simulink model "DSB_AMwithAWGN"  (R2018a)
settings: Solver=VariableStepAuto  StartTime=0.0  StopTime=0.005  RelTol=1e-3
libraries: commchan3 x1, dsparch4 x1
settings Model: Creator=Neo  LastModifiedBy=Neo

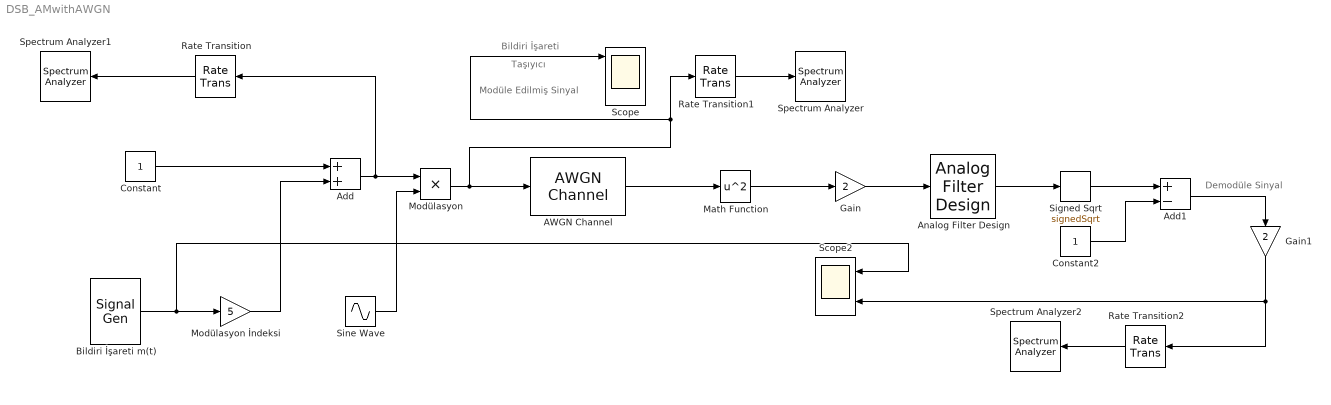
== system DSB_AMwithAWGN ==
  note: Demodüle Sinyal
  note: Modüle Edilmiş Sinyal
  note: Taşıyıcı
  note: Bildiri İşareti
  AWGN Channel : commchan3/AWGN Channel  InputProcessing=Columns as channels (frame based)  seed=67  noiseMode=Variance from mask  EbNodB=10  EsNodB=10  SNRdB=10  bitsPerSym=1  Ps=1  Tsym=1  variance=0.5
  Add : Sum
  Add1 : Sum  Inputs=+-
  Analog Filter Design : dsparch4/Analog Filter Design  method=Butterworth  filttype=Lowpass  N=100  Wlo=2*pi*5000  Whi=80  Rp=2  Rs=40
  Bildiri İşareti m(t) : SignalGenerator  Frequency=1000
  Constant : Constant
  Constant2 : Constant
  Gain : Gain  Gain=2
  "Gain1 " : Gain  Gain=2
  Math Function : Math  Operator=square  SaturateOnIntegerOverflow=on
  Modülasyon : Product
  Modülasyon İndeksi : Gain  Gain=5
  Rate Transition : RateTransition  OutPortSampleTime=1/8e4
  Rate Transition1 : RateTransition  OutPortSampleTime=1/8e4
  Rate Transition2 : RateTransition  OutPortSampleTime=1/8e4
  Scope : Scope  NumInputPorts=3
  Scope2 : Scope  NumInputPorts=2
  Signed Sqrt : Sqrt  Operator=signedSqrt  SaturateOnIntegerOverflow=on
  Sine Wave : Sin  Frequency=2*pi*10000  Phase=pi/2  SampleTime=0
  Spectrum Analyzer : SpectrumAnalyzer
  Spectrum Analyzer1 : SpectrumAnalyzer
  Spectrum Analyzer2 : SpectrumAnalyzer
  wires:
  Modülasyon İndeksi/1 -> Add/2
  Add/1 -> Rate Transition/1, Modülasyon/1
  Constant/1 -> Add/1
  Rate Transition1/1 -> Spectrum Analyzer/1
  Bildiri İşareti m(t)/1 -> Modülasyon İndeksi/1, Scope2/1
  Rate Transition/1 -> Spectrum Analyzer1/1
  Sine Wave/1 -> Modülasyon/2
  Math Function/1 -> Gain/1
  Gain/1 -> Analog Filter Design/1
  Analog Filter Design/1 -> Signed Sqrt/1
  Signed Sqrt/1 -> Add1/1
  Constant2/1 -> Add1/2
  Add1/1 -> "Gain1 "/1
  "Gain1 "/1 -> Scope2/2, Rate Transition2/1
  Rate Transition2/1 -> Spectrum Analyzer2/1
  Modülasyon/1 -> AWGN Channel/1, Rate Transition1/1, Scope/1
  AWGN Channel/1 -> Math Function/1
